simulink model "1_ViertelFzg"  (R2016a)
settings: Solver=ode4  StartTime=t_start  StopTime=t_end  FixedStep=h  RelTol=1e-3
values from neighbouring files (symbols this model uses):
  c_suspension = setting(i,3)    [1_ViertelFzg_Parameters.m]
  c_tire = setting(i,5)    [1_ViertelFzg_Parameters.m]
  d_suspension = setting(i,4)    [1_ViertelFzg_Parameters.m]
  m_vehicle_body = setting(i,2)    [1_ViertelFzg_Parameters.m]
  m_wheel_body = setting(i,6)    [1_ViertelFzg_Parameters.m]
  z1_0 = -((m_vehicle_body+m_wheel_body)*9.81)/c_tire    (= -0.016455483871)    [1_ViertelFzg_Parameters.m]
  z2_0 = z1_0 - m_vehicle_body*9.81/c_suspension    (= -0.278055483871)    [1_ViertelFzg_Parameters.m]
undefined symbols (not defined in the file or in its folder): z_A_max
settings Model: Creator=KFZ00  LastModifiedBy=Dominik
settings DataIOCC: SaveOutput=off  TimeSaveName=t_out
settings DebuggingCC: AllowSymbolicDim=off
settings ModelReferenceCC: PropagateSignalLabelsOutOfModel=off
settings GRTTargetCC: GeneratePreprocessorConditionals=Use local settings

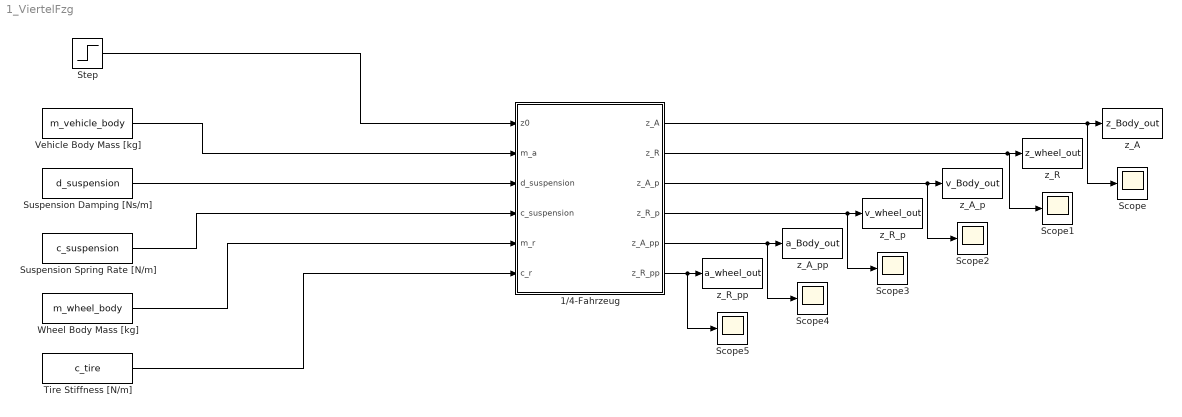
== system 1_ViertelFzg ==
  1/4-Fahrzeug : Subsystem
  Scope{,1..5} (6 alike) : Scope
  Step : Step  Time=0.5  After=0.02  SampleTime=0
  Suspension Damping [Ns/m] : Constant  Value=d_suspension
  Suspension Spring Rate [N/m] : Constant  Value=c_suspension
  Tire Stiffness [N/m] : Constant  Value=c_tire
  Vehicle Body Mass [kg] : Constant  Value=m_vehicle_body
  Wheel Body Mass [kg] : Constant  Value=m_wheel_body
  z_A : ToWorkspace  VariableName=z_Body_out  SampleTime=-1
      settings: Save2DSignal=2-D array (concatenate along first dimension)
  z_A_p : ToWorkspace  VariableName=v_Body_out  SampleTime=-1
      settings: Save2DSignal=2-D array (concatenate along first dimension)
  z_A_pp : ToWorkspace  VariableName=a_Body_out  SampleTime=-1
      settings: Save2DSignal=2-D array (concatenate along first dimension)
  z_R : ToWorkspace  VariableName=z_wheel_out  SampleTime=-1
      settings: Save2DSignal=2-D array (concatenate along first dimension)
  z_R_p : ToWorkspace  VariableName=v_wheel_out  SampleTime=-1
      settings: Save2DSignal=2-D array (concatenate along first dimension)
  z_R_pp : ToWorkspace  VariableName=a_wheel_out  SampleTime=-1
      settings: Save2DSignal=2-D array (concatenate along first dimension)
  wires:
  Tire Stiffness [N/m]/1 -> 1/4-Fahrzeug/6(c_r)
  Wheel Body Mass [kg]/1 -> 1/4-Fahrzeug/5(m_r)
  Vehicle Body Mass [kg]/1 -> 1/4-Fahrzeug/2(m_a)
  Suspension Spring Rate [N/m]/1 -> 1/4-Fahrzeug/4(c_suspension)
  Suspension Damping [Ns/m]/1 -> 1/4-Fahrzeug/3(d_suspension)
  Step/1 -> 1/4-Fahrzeug/1(z0)
  1/4-Fahrzeug/1(z_A) -> Scope/1, z_A/1
  1/4-Fahrzeug/2(z_R) -> Scope1/1, z_R/1
  1/4-Fahrzeug/3(z_A_p) -> Scope2/1, z_A_p/1
  1/4-Fahrzeug/4(z_R_p) -> Scope3/1, z_R_p/1
  1/4-Fahrzeug/6(z_R_pp) -> Scope5/1, z_R_pp/1
  1/4-Fahrzeug/5(z_A_pp) -> Scope4/1, z_A_pp/1

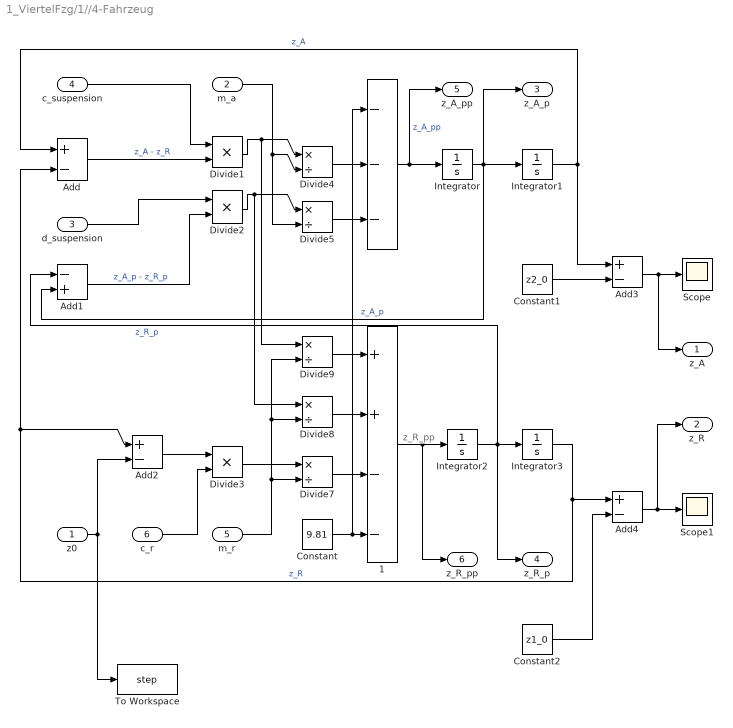
== system 1_ViertelFzg/1//4-Fahrzeug ==
  note: z_R_pp
  z0 : Inport
  m_a : Inport  Port=2
  d_suspension : Inport  Port=3
  c_suspension : Inport  Port=4
  m_r : Inport  Port=5
  c_r : Inport  Port=6
  " " : Sum  Inputs=---
  1 : Sum  Inputs=++--
  Add{,2..4} (4 alike) : Sum  Inputs=+-
  Add1 : Sum  Inputs=-+
  Constant : Constant  Value=9.81
  Constant1 : Constant  Value=z2_0
  Constant2 : Constant  Value=z1_0
  Divide1 : Product  Inputs=**
  Divide2 : Product  Inputs=**
  Divide3 : Product  Inputs=**
  Divide{4..5,7..9} (5 alike) : Product  Inputs=*/
  Integrator : Integrator
  Integrator1 : Integrator  InitialCondition=z2_0  UpperSaturationLimit=z_A_max  LowerSaturationLimit=-z_A_max
  Integrator2 : Integrator
  Integrator3 : Integrator  InitialCondition=z1_0
  Scope : Scope
  Scope1 : Scope
  To Workspace : ToWorkspace  VariableName=step  SampleTime=-1
      settings: Save2DSignal=2-D array (concatenate along first dimension)
  z_A : Outport
  z_R : Outport  Port=2
  z_A_p : Outport  Port=3
  z_R_p : Outport  Port=4
  z_A_pp : Outport  Port=5
  z_R_pp : Outport  Port=6
  wires:
  Integrator1/1 -> Add3/1, Add/1  "z_A"
  1/1 -> Integrator2/1, z_R_pp/1
  Divide7/1 -> 1/3
  Divide5/1 -> " "/3
  Integrator3/1 -> Add/2, Add2/1, Add4/1  "z_R"
  Divide9/1 -> 1/1
  c_suspension/1 -> Divide1/1
  " "/1 -> z_A_pp/1, Integrator/1  "z_A_pp"
  Divide2/1 -> Divide8/1, Divide5/1
  Integrator/1 -> z_A_p/1, Integrator1/1, Add1/2  "z_A_p"
  Divide4/1 -> " "/2
  Divide1/1 -> Divide9/1, Divide4/1
  Add2/1 -> Divide3/1
  z0/1 -> Add2/2, To Workspace/1
  Divide8/1 -> 1/2
  Constant/1 -> " "/1, 1/4
  Divide3/1 -> Divide7/1
  m_r/1 -> Divide9/2, Divide8/2, Divide7/2
  Add/1 -> Divide1/2  "z_A - z_R"
  Integrator2/1 -> z_R_p/1, Add1/1, Integrator3/1  "z_R_p"
  Add1/1 -> Divide2/2  "z_A_p - z_R_p"
  d_suspension/1 -> Divide2/1
  m_a/1 -> Divide5/2, Divide4/2
  c_r/1 -> Divide3/2
  Constant1/1 -> Add3/2
  Add3/1 -> Scope/1, z_A/1
  Constant2/1 -> Add4/2
  Add4/1 -> z_R/1, Scope1/1
